simulink model "BLDC_dq_Control_Gradual"  (R2021a)
settings: Solver=FixedStepAuto  StartTime=0.0  StopTime=12  FixedStep=0.000002  RelTol=1e-3
model workspace (MAT data in the model file):
  Tl = 3
undefined symbols (not defined in the file): sigbuilder_block
libraries: pid_lib x9, spsMosfetLib x6, spsVoltageMeasurementLib x3, simulink x2, spsDCVoltageSourceLib x1, spspowerguiLib x1
(part 2 of 2)

== matlab function BLDC_dq_Control_Gradual/InvParkClarke1 ==
  data: X_dq input; Y_abc output; theta input
function Y_abc = fcn(X_dq, theta)
X_dq0 = [X_dq;0];

%inverse Park-Clarke power invariant
iT_PC = sqrt(2/3)*[cos(theta)          -sin(theta)            1/sqrt(2); ...
                  cos(theta-2*pi/3)   -sin(theta-2*pi/3)     1/sqrt(2); ...
                  cos(theta+2*pi/3)   -sin(theta+2*pi/3)     1/sqrt(2)];
%               
              
 %inverse Park-Clarke amplitude invariant
% iT_PC = [cos(theta)          -sin(theta)            1; ...
%          cos(theta-2*pi/3)   -sin(theta-2*pi/3)     1; ...
%          cos(theta+2*pi/3)   -sin(theta+2*pi/3)     1];



Y_abc =iT_PC*X_dq0;
end

== matlab function BLDC_dq_Control_Gradual/ParkClarke ==
  data: X_abc input; Y_dq output; theta input
function Y_dq = fcn(X_abc, theta)

% Park clarke transform eliminating the third element
PC_T = (sqrt(2)/2)*[sqrt(3)*cos(theta)  sin(theta)  -sin(theta) ; ...
                    -sqrt(3)*sin(theta)  cos(theta)  -cos(theta)];

Y_dq =PC_T*X_abc;
end
